simulink library "Flow_Mixer_Thermostatic"  (Simulink 8.2)
settings: Solver=ode45  StartTime=0.0  StopTime=10.0  RelTol=1e-3
libraries: simulink x2, carnot x1
settings Model: Creator=lena.frank  LastModifiedBy=drhf

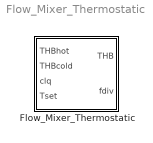
== system Flow_Mixer_Thermostatic ==
  Flow_Mixer_Thermostatic : Subsystem  mask(thermostatic flow mixer){t=10}
      mask prompts: t "time constant for valve [s]"
      mask help:
      | The thermostatic flow mixer mixes cold and hot fluid to set a desired temperature and calculates the pressure drop.
      | Use together with flow_diverter_fixed_rate.
      mask init:
      | if t < 0.01
      |     t = 0.01;
      |     disp('Flow mixer thermostatic: time constant set to minimum value 0.01')
      | end
      | t1 = 1/t;
      mask Help: web(fullfile(path_carnot('help'),'Flow_Mixer.html'),'-helpbrowser')
      mask Display: plot(10,0,100,100,[40,60,60,40,40],[60,40,60,40,60],[44,50,56,44],[66,50,66,66],[50,50],[30,50],[56,44],[25,25],[50,50],[10,25])

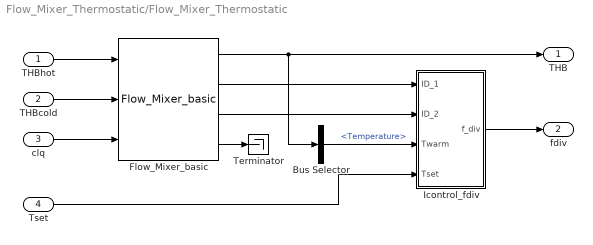
== system Flow_Mixer_Thermostatic/Flow_Mixer_Thermostatic ==
  THBhot : Inport
  THBcold : Inport  Port=2
  clq : Inport  Port=3
  Tset : Inport  Port=4
  Bus Selector : BusSelector  OutputSignals=Temperature
  Flow_Mixer_basic : carnot/Basic/Hydraulics/Flow_Mixer_basic
  Icontrol_fdiv : Subsystem
  Terminator : Terminator
  THB : Outport
  fdiv : Outport  Port=2
  wires:
  Icontrol_fdiv/1(f_div) -> fdiv/1
  THBhot/1 -> Flow_Mixer_basic/1
  THBcold/1 -> Flow_Mixer_basic/2
  clq/1 -> Flow_Mixer_basic/3
  Flow_Mixer_basic/1 -> THB/1, Bus Selector/1
  Flow_Mixer_basic/2 -> Icontrol_fdiv/1(ID_1)
  Flow_Mixer_basic/3 -> Icontrol_fdiv/2(ID_2)
  Tset/1 -> Icontrol_fdiv/4(Tset)
  Flow_Mixer_basic/4 -> Terminator/1
  Bus Selector/1 -> Icontrol_fdiv/3(Twarm)  "<Temperature>"

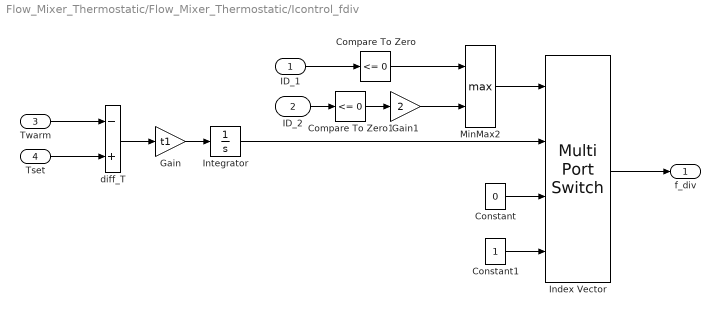
== system Flow_Mixer_Thermostatic/Flow_Mixer_Thermostatic/Icontrol_fdiv ==
  ID_1 : Inport
  ID_2 : Inport  Port=2
  Twarm : Inport  Port=3
  Tset : Inport  Port=4
  Compare To Zero : simulink/Logic and Bit Operations/Compare To Zero  relop=<=  OutDataTypeStr=uint8
  Compare To Zero1 : simulink/Logic and Bit Operations/Compare To Zero  relop=<=  OutDataTypeStr=uint8
  Constant : Constant  Value=0
  Constant1 : Constant
  Gain : Gain  Gain=t1  SaturateOnIntegerOverflow=on  OutDataTypeStr=Inherit: Same as input  ParamDataTypeStr=Inherit: Same as input
  Gain1 : Gain  Gain=2
  Index Vector : MultiPortSwitch  DataPortOrder=Zero-based contiguous  zeroidx=on
  Integrator : Integrator  LimitOutput=on  UpperSaturationLimit=1  LowerSaturationLimit=0
  MinMax2 : MinMax  Function=max  Inputs=2
  diff_T : Sum  Inputs=-+  SaturateOnIntegerOverflow=on  InputSameDT=on  OutDataTypeStr=Inherit: Same as first input
  f_div : Outport
  wires:
  Compare To Zero1/1 -> Gain1/1
  Compare To Zero/1 -> MinMax2/1
  MinMax2/1 -> Index Vector/1
  ID_1/1 -> Compare To Zero/1
  ID_2/1 -> Compare To Zero1/1
  Constant/1 -> Index Vector/3
  Integrator/1 -> Index Vector/2
  Constant1/1 -> Index Vector/4
  Gain1/1 -> MinMax2/2
  Index Vector/1 -> f_div/1
  Tset/1 -> diff_T/2
  Twarm/1 -> diff_T/1
  Gain/1 -> Integrator/1
  diff_T/1 -> Gain/1
